simulink model "symulacja_OL"  (R2019b)
settings: Solver=VariableStepAuto  StartTime=0.0  StopTime=50  RelTol=1e-3
values from neighbouring files (symbols this model uses):
  d = 1    [lab8.m]
  K = 0.16*Ku    [lab8.m]
  Ki = 1/Ti    (= 1e-10)    [lab8.m]
  m = 0.5    [lab8.m]
  T_o = 0.1    [lab8.m]
  Td = ((0.15*(1-kappa))*Tu)/(1-0.95*kappa)    [lab8.m]
settings Model: Creator=kacpe  LastModifiedBy=kacpe

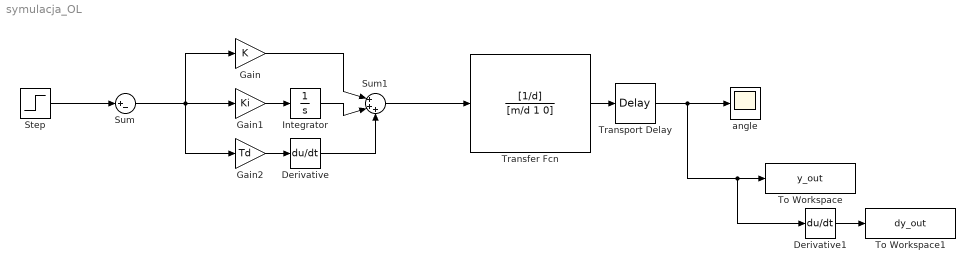
== system symulacja_OL ==
  Derivative : Derivative
  Derivative1 : Derivative
  Gain : Gain  Gain=K
  Gain1 : Gain  Gain=Ki
  Gain2 : Gain  Gain=Td
  Integrator : Integrator
  Step : Step  SampleTime=0
  Sum : Sum  Inputs=|+-
  Sum1 : Sum  Inputs=|+++
  To Workspace : ToWorkspace  VariableName=y_out  SampleTime=-1
  To Workspace1 : ToWorkspace  VariableName=dy_out  SampleTime=-1
  Transfer Fcn : TransferFcn  Numerator=[1/d]  Denominator=[m/d 1 0]
  Transport Delay : TransportDelay  DelayTime=T_o
  "angle " : Scope
  wires:
  Step/1 -> Sum/1
  Sum/1 -> Gain/1, Gain2/1, Gain1/1
  Gain1/1 -> Integrator/1
  Gain2/1 -> Derivative/1
  Gain/1 -> Sum1/1
  Sum1/1 -> Transfer Fcn/1
  Transfer Fcn/1 -> Transport Delay/1
  Transport Delay/1 -> Derivative1/1, To Workspace/1, "angle "/1
  Derivative1/1 -> To Workspace1/1
  Integrator/1 -> Sum1/2
  Derivative/1 -> Sum1/3
